simulink model "DR18E_Testpult"  (R2017a)
settings: Solver=ode1  StartTime=0.0  StopTime=Inf  FixedStep=0.001  RelTol=1e-3
PostLoadFcn:
  | , if any(exist('dsrtsu_mdlpostloadfcn', 'file') == [2, 3, 6]), try dsrtsu_mdlpostloadfcn('Execute', bdroot); catch fprintf('Error in PostLoadFcn (dsrtsu_mdlpostloadfcn) for model "%s":\n %s\n', bdroot, lasterr); end, end,
model workspace: external: MATLAB File C:\Users\DeltaRacing\Documents\dSPACE\MABX_DR18E\Model\DR18E_MABX_Parameter.m (data not in the file)
values from neighbouring files (symbols this model uses):
  am = 1/Ts    (= 1)    [DR18E_MABX_Parameter.m]
  bm = K/Ts    (= 0.05)    [DR18E_MABX_Parameter.m]
  cf = 41350    [DR18E_MABX_Parameter.m]
  cr = 41350    [DR18E_MABX_Parameter.m]
  Derating_HV_Battery_Kapa = 1    [DR18E_MABX_Parameter.m]
  Derating_Start_km = 16    [DR18E_MABX_Parameter.m]
  Drive_Mode = 0    [DR18E_MABX_Parameter.m]
  g = 1    [DR18E_MABX_Parameter.m]
  Gas_Modus = 2    [DR18E_MABX_Parameter.m]
  HV_Power_max = 80    [DR18E_MABX_Parameter.m]
  i_Getriebe = 3.3    [DR18E_MABX_Parameter.m]
  i_Lenkgetriebe = 4.32    [DR18E_MABX_Parameter.m]
  K_SET = 1    [DR18E_MABX_Parameter.m]
  Kapazitaet_HV_Battery_kWh = 6.6    [DR18E_MABX_Parameter.m]
  KW_T_Soll = 37    [DR18E_MABX_Parameter.m]
  lf = 1.2    [DR18E_MABX_Parameter.m]
  lr = 1.15    [DR18E_MABX_Parameter.m]
  m = 310    [DR18E_MABX_Parameter.m]
  M_max = 150    [DR18E_MABX_Parameter.m]
  Power_Limit_onoff = 0    [DR18E_MABX_Parameter.m]
  Reifenradius = 0.2351    [DR18E_MABX_Parameter.m]
  Strecke_Endu_km = 22    [DR18E_MABX_Parameter.m]
  TC_Decr_Gas = 0.00005    (= 5e-05)    [DR18E_MABX_Parameter.m]
  TC_Derivative = 0.4    [DR18E_MABX_Parameter.m]
  TC_Incr_Gas = 0.005    [DR18E_MABX_Parameter.m]
  TC_On = 0    [DR18E_MABX_Parameter.m]
  TC_Relay_Off = 0.065    [DR18E_MABX_Parameter.m]
  TC_Relay_On = 0.07    [DR18E_MABX_Parameter.m]
  TV_Mode = 2    [DR18E_MABX_Parameter.m]
  TV_On = 0    [DR18E_MABX_Parameter.m]
  TV_Override = 1    [DR18E_MABX_Parameter.m]
  y = 0.8    [DR18E_MABX_Parameter.m]
undefined symbols (not defined in the file or in its folder): D, DiscIntNeverNeededParam, I, K_OL, P
libraries: simulink x288, rtican x105, rtiusbflightreclib x40, rti1401lib_dio_type3 x10, simulink_extras x10, rti1401lib_adc_type4 x8, rti1401lib_II_base x7
(part 17 of 28)

== system DR18E_Testpult/Eingabe Fahrzeug/MicroAutoBox/Beschleunigungssensor ==
  Bus Creator : BusCreator  Inputs=3
  DS1401_ACCEL_READ_BL1 : rti1401lib_II_base/DS1401_ACCEL_READ_BL1  DSProperties=struct('RTI',struct('Version',uint32(1),'BlockType',struct('isSLSource',uint8(1),'isSLSink',uint8(0),'isHWSource',uint8(1),'isHWSink',uint8(0),'isSetup',uint8(0),'isInline',uint8(1),'isNonInline',uint8(0),'isInterrupt',uint8(0),'isChannelwise',uint8(0)),'IOBoardType',{{'DS1401','BASE','II'}},'UnitType','ACCEL','Identifier','ACCELREAD','DialogType','ML','BlockSet','NONE','SlaveProcessor','NONE'))  RTIBlockInterface=struct('OutputPortsWidth',int32([1 1 1 1]),'OutputPortsActive',[1 1 1 1],'OutputPortsDataType',{{'SS_UINT32','SS_DOUBLE','SS_DOUBLE','SS_DOUBLE'}},'OutputPortsName',{{'Count','X','Y','Z'}},'BlockDisplay',{{'Acceleration\nSensor','center'}},'IconTransparency','on','InitLevel',3,'DialogFcn','rti1401baseiiaccelreadgui','BlockName',struct('Token',{{'DS1401_ACCEL_READ_BL1'}}))  RTIBlockParameters=struct('SampleRate',{{5,'OFF',[1 8]}},'ReadMode',{{1,'OFF',[1 2]}},'SensorRange',{{3,'OFF',[1 3]}},'TLCFileName',{{'rti1401base_II_accel_read','OFF',[]}})  RTISFcnParameters=struct('SampleRate','int16','ReadMode','int16','SensorRange','int16','TLCFileName','char')  RTIBlockParaDefault=struct('SampleRate',3,'ReadMode',1,'SensorRange',1,'TLCFileName','rti1401base_II_accel_read')
  Beschleunigungssensor : Outport
  wires:
  Bus Creator/1 -> Beschleunigungssensor/1  "Beschleunigungssensor"
  DS1401_ACCEL_READ_BL1/2 -> Bus Creator/1  "x"
  DS1401_ACCEL_READ_BL1/3 -> Bus Creator/2  "y"
  DS1401_ACCEL_READ_BL1/4 -> Bus Creator/3  "z"

== system DR18E_Testpult/Eingabe Fahrzeug/MicroAutoBox/DI ==
  note: Direct DI
  note: Soundboard
  Bus Creator : BusCreator  Inputs=11
  DIO_TYPE3_BIT_IN_CH_BL1 : rti1401lib_dio_type3/DIO_TYPE3_BIT_IN_CH_BL1  DSProperties=struct('RTI',struct('Version',uint32(2),'BlockType',struct('isSLSource',uint8(1),'isSLSink',uint8(0),'isHWSource',uint8(1),'isHWSink',uint8(0),'isSetup',uint8(0),'isInline',uint8(1),'isNonInline',uint8(0),'isInterrupt',uint8(0),'isChannelwise',uint8(1)),'IOBoardType',{{'DS1401','STD','DIOT3'}},'UnitType','BIT','Identifier','BITINCH','DialogType','ML','BlockSet','NONE','SlaveProcessor','NONE'))  RTIBlockInterface=struct('OutputPortsWidth',int32(1),'OutputPortsDataType',{{'SS_BOOLEAN'}},'OutputPortsActive',1,'OutputPortsName',{{'Out'}},'BlockDisplay',{{['DIO TP3 BIT IN\n Channelwise\nModule: 1\nPort: 2\nChannel: 1'],'center'}},'IconTransparency','on','InitLevel',3,'DialogFcn','rti1401stddiot3bitinchgui','BlockName',struct('Token',{{'DIO_TYPE3_BIT_IN_CH_BL1'}}))  RTIBlockParameters=struct('ModuleNo',{{1,'OFF',[1 16]}},'PortNo',{{2,'OFF',[1 3]}},'ChannelNo',{{1,'OFF',[1 16]}},'TLCFileName',{{'rti1401dio_t3_bit_in_ch','OFF',[]}},'EnableInterrupt',{{0,'OFF',[0 1]}},'TriggerEdgeType',{{1,'OFF',[1 3]}})  RTISFcnParameters=struct('ModuleNo','int32','PortNo','int16','ChannelNo','int16','TLCFileName','char','EnableInterrupt','int16','TriggerEdgeType','int32')  RTIBlockParaDefault=struct('ModuleNo',1,'PortNo',1,'ChannelNo',1,'TLCFileName','rti1401dio_t3_bit_in_ch','EnableInterrupt',0,'TriggerEdgeType',1)
  DIO_TYPE3_BIT_IN_CH_BL10 : rti1401lib_dio_type3/DIO_TYPE3_BIT_IN_CH_BL1  DSProperties=struct('RTI',struct('Version',uint32(2),'BlockType',struct('isSLSource',uint8(1),'isSLSink',uint8(0),'isHWSource',uint8(1),'isHWSink',uint8(0),'isSetup',uint8(0),'isInline',uint8(1),'isNonInline',uint8(0),'isInterrupt',uint8(0),'isChannelwise',uint8(1)),'IOBoardType',{{'DS1401','STD','DIOT3'}},'UnitType','BIT','Identifier','BITINCH','DialogType','ML','BlockSet','NONE','SlaveProcessor','NONE'))  RTIBlockInterface=struct('OutputPortsWidth',int32(1),'OutputPortsDataType',{{'SS_BOOLEAN'}},'OutputPortsActive',1,'OutputPortsName',{{'Out'}},'BlockDisplay',{{['DIO TP3 BIT IN\n Channelwise\nModule: 1\nPort: 2\nChannel: 11'],'center'}},'IconTransparency','on','InitLevel',3,'DialogFcn','rti1401stddiot3bitinchgui','BlockName',struct('Token',{{'DIO_TYPE3_BIT_IN_CH_BL1'}}))  RTIBlockParameters=struct('ModuleNo',{{1,'OFF',[1 16]}},'PortNo',{{2,'OFF',[1 3]}},'ChannelNo',{{11,'OFF',[1 16]}},'TLCFileName',{{'rti1401dio_t3_bit_in_ch','OFF',[]}},'EnableInterrupt',{{0,'OFF',[0 1]}},'TriggerEdgeType',{{1,'OFF',[1 3]}})  RTISFcnParameters=struct('ModuleNo','int32','PortNo','int16','ChannelNo','int16','TLCFileName','char','EnableInterrupt','int16','TriggerEdgeType','int32')  RTIBlockParaDefault=struct('ModuleNo',1,'PortNo',1,'ChannelNo',1,'TLCFileName','rti1401dio_t3_bit_in_ch','EnableInterrupt',0,'TriggerEdgeType',1)
  DIO_TYPE3_BIT_IN_CH_BL2 : rti1401lib_dio_type3/DIO_TYPE3_BIT_IN_CH_BL1  DSProperties=struct('RTI',struct('Version',uint32(2),'BlockType',struct('isSLSource',uint8(1),'isSLSink',uint8(0),'isHWSource',uint8(1),'isHWSink',uint8(0),'isSetup',uint8(0),'isInline',uint8(1),'isNonInline',uint8(0),'isInterrupt',uint8(0),'isChannelwise',uint8(1)),'IOBoardType',{{'DS1401','STD','DIOT3'}},'UnitType','BIT','Identifier','BITINCH','DialogType','ML','BlockSet','NONE','SlaveProcessor','NONE'))  RTIBlockInterface=struct('OutputPortsWidth',int32(1),'OutputPortsDataType',{{'SS_BOOLEAN'}},'OutputPortsActive',1,'OutputPortsName',{{'Out'}},'BlockDisplay',{{['DIO TP3 BIT IN\n Channelwise\nModule: 1\nPort: 2\nChannel: 2'],'center'}},'IconTransparency','on','InitLevel',3,'DialogFcn','rti1401stddiot3bitinchgui','BlockName',struct('Token',{{'DIO_TYPE3_BIT_IN_CH_BL1'}}))  RTIBlockParameters=struct('ModuleNo',{{1,'OFF',[1 16]}},'PortNo',{{2,'OFF',[1 3]}},'ChannelNo',{{2,'OFF',[1 16]}},'TLCFileName',{{'rti1401dio_t3_bit_in_ch','OFF',[]}},'EnableInterrupt',{{0,'OFF',[0 1]}},'TriggerEdgeType',{{1,'OFF',[1 3]}})  RTISFcnParameters=struct('ModuleNo','int32','PortNo','int16','ChannelNo','int16','TLCFileName','char','EnableInterrupt','int16','TriggerEdgeType','int32')  RTIBlockParaDefault=struct('ModuleNo',1,'PortNo',1,'ChannelNo',1,'TLCFileName','rti1401dio_t3_bit_in_ch','EnableInterrupt',0,'TriggerEdgeType',1)
  DIO_TYPE3_BIT_IN_CH_BL3 : rti1401lib_dio_type3/DIO_TYPE3_BIT_IN_CH_BL1  DSProperties=struct('RTI',struct('Version',uint32(2),'BlockType',struct('isSLSource',uint8(1),'isSLSink',uint8(0),'isHWSource',uint8(1),'isHWSink',uint8(0),'isSetup',uint8(0),'isInline',uint8(1),'isNonInline',uint8(0),'isInterrupt',uint8(0),'isChannelwise',uint8(1)),'IOBoardType',{{'DS1401','STD','DIOT3'}},'UnitType','BIT','Identifier','BITINCH','DialogType','ML','BlockSet','NONE','SlaveProcessor','NONE'))  RTIBlockInterface=struct('OutputPortsWidth',int32(1),'OutputPortsDataType',{{'SS_BOOLEAN'}},'OutputPortsActive',1,'OutputPortsName',{{'Out'}},'BlockDisplay',{{['DIO TP3 BIT IN\n Channelwise\nModule: 1\nPort: 2\nChannel: 6'],'center'}},'IconTransparency','on','InitLevel',3,'DialogFcn','rti1401stddiot3bitinchgui','BlockName',struct('Token',{{'DIO_TYPE3_BIT_IN_CH_BL1'}}))  RTIBlockParameters=struct('ModuleNo',{{1,'OFF',[1 16]}},'PortNo',{{2,'OFF',[1 3]}},'ChannelNo',{{6,'OFF',[1 16]}},'TLCFileName',{{'rti1401dio_t3_bit_in_ch','OFF',[]}},'EnableInterrupt',{{0,'OFF',[0 1]}},'TriggerEdgeType',{{1,'OFF',[1 3]}})  RTISFcnParameters=struct('ModuleNo','int32','PortNo','int16','ChannelNo','int16','TLCFileName','char','EnableInterrupt','int16','TriggerEdgeType','int32')  RTIBlockParaDefault=struct('ModuleNo',1,'PortNo',1,'ChannelNo',1,'TLCFileName','rti1401dio_t3_bit_in_ch','EnableInterrupt',0,'TriggerEdgeType',1)
  DIO_TYPE3_BIT_IN_CH_BL4 : rti1401lib_dio_type3/DIO_TYPE3_BIT_IN_CH_BL1  DSProperties=struct('RTI',struct('Version',uint32(2),'BlockType',struct('isSLSource',uint8(1),'isSLSink',uint8(0),'isHWSource',uint8(1),'isHWSink',uint8(0),'isSetup',uint8(0),'isInline',uint8(1),'isNonInline',uint8(0),'isInterrupt',uint8(0),'isChannelwise',uint8(1)),'IOBoardType',{{'DS1401','STD','DIOT3'}},'UnitType','BIT','Identifier','BITINCH','DialogType','ML','BlockSet','NONE','SlaveProcessor','NONE'))  RTIBlockInterface=struct('OutputPortsWidth',int32(1),'OutputPortsDataType',{{'SS_BOOLEAN'}},'OutputPortsActive',1,'OutputPortsName',{{'Out'}},'BlockDisplay',{{['DIO TP3 BIT IN\n Channelwise\nModule: 1\nPort: 2\nChannel: 4'],'center'}},'IconTransparency','on','InitLevel',3,'DialogFcn','rti1401stddiot3bitinchgui','BlockName',struct('Token',{{'DIO_TYPE3_BIT_IN_CH_BL1'}}))  RTIBlockParameters=struct('ModuleNo',{{1,'OFF',[1 16]}},'PortNo',{{2,'OFF',[1 3]}},'ChannelNo',{{4,'OFF',[1 16]}},'TLCFileName',{{'rti1401dio_t3_bit_in_ch','OFF',[]}},'EnableInterrupt',{{0,'OFF',[0 1]}},'TriggerEdgeType',{{1,'OFF',[1 3]}})  RTISFcnParameters=struct('ModuleNo','int32','PortNo','int16','ChannelNo','int16','TLCFileName','char','EnableInterrupt','int16','TriggerEdgeType','int32')  RTIBlockParaDefault=struct('ModuleNo',1,'PortNo',1,'ChannelNo',1,'TLCFileName','rti1401dio_t3_bit_in_ch','EnableInterrupt',0,'TriggerEdgeType',1)
  DIO_TYPE3_BIT_IN_CH_BL5 : rti1401lib_dio_type3/DIO_TYPE3_BIT_IN_CH_BL1  DSProperties=struct('RTI',struct('Version',uint32(2),'BlockType',struct('isSLSource',uint8(1),'isSLSink',uint8(0),'isHWSource',uint8(1),'isHWSink',uint8(0),'isSetup',uint8(0),'isInline',uint8(1),'isNonInline',uint8(0),'isInterrupt',uint8(0),'isChannelwise',uint8(1)),'IOBoardType',{{'DS1401','STD','DIOT3'}},'UnitType','BIT','Identifier','BITINCH','DialogType','ML','BlockSet','NONE','SlaveProcessor','NONE'))  RTIBlockInterface=struct('OutputPortsWidth',int32(1),'OutputPortsDataType',{{'SS_BOOLEAN'}},'OutputPortsActive',1,'OutputPortsName',{{'Out'}},'BlockDisplay',{{['DIO TP3 BIT IN\n Channelwise\nModule: 1\nPort: 2\nChannel: 5'],'center'}},'IconTransparency','on','InitLevel',3,'DialogFcn','rti1401stddiot3bitinchgui','BlockName',struct('Token',{{'DIO_TYPE3_BIT_IN_CH_BL1'}}))  RTIBlockParameters=struct('ModuleNo',{{1,'OFF',[1 16]}},'PortNo',{{2,'OFF',[1 3]}},'ChannelNo',{{5,'OFF',[1 16]}},'TLCFileName',{{'rti1401dio_t3_bit_in_ch','OFF',[]}},'EnableInterrupt',{{0,'OFF',[0 1]}},'TriggerEdgeType',{{1,'OFF',[1 3]}})  RTISFcnParameters=struct('ModuleNo','int32','PortNo','int16','ChannelNo','int16','TLCFileName','char','EnableInterrupt','int16','TriggerEdgeType','int32')  RTIBlockParaDefault=struct('ModuleNo',1,'PortNo',1,'ChannelNo',1,'TLCFileName','rti1401dio_t3_bit_in_ch','EnableInterrupt',0,'TriggerEdgeType',1)
  DIO_TYPE3_BIT_IN_CH_BL6 : rti1401lib_dio_type3/DIO_TYPE3_BIT_IN_CH_BL1  DSProperties=struct('RTI',struct('Version',uint32(2),'BlockType',struct('isSLSource',uint8(1),'isSLSink',uint8(0),'isHWSource',uint8(1),'isHWSink',uint8(0),'isSetup',uint8(0),'isInline',uint8(1),'isNonInline',uint8(0),'isInterrupt',uint8(0),'isChannelwise',uint8(1)),'IOBoardType',{{'DS1401','STD','DIOT3'}},'UnitType','BIT','Identifier','BITINCH','DialogType','ML','BlockSet','NONE','SlaveProcessor','NONE'))  RTIBlockInterface=struct('OutputPortsWidth',int32(1),'OutputPortsDataType',{{'SS_BOOLEAN'}},'OutputPortsActive',1,'OutputPortsName',{{'Out'}},'BlockDisplay',{{['DIO TP3 BIT IN\n Channelwise\nModule: 1\nPort: 2\nChannel: 8'],'center'}},'IconTransparency','on','InitLevel',3,'DialogFcn','rti1401stddiot3bitinchgui','BlockName',struct('Token',{{'DIO_TYPE3_BIT_IN_CH_BL1'}}))  RTIBlockParameters=struct('ModuleNo',{{1,'OFF',[1 16]}},'PortNo',{{2,'OFF',[1 3]}},'ChannelNo',{{8,'OFF',[1 16]}},'TLCFileName',{{'rti1401dio_t3_bit_in_ch','OFF',[]}},'EnableInterrupt',{{0,'OFF',[0 1]}},'TriggerEdgeType',{{1,'OFF',[1 3]}})  RTISFcnParameters=struct('ModuleNo','int32','PortNo','int16','ChannelNo','int16','TLCFileName','char','EnableInterrupt','int16','TriggerEdgeType','int32')  RTIBlockParaDefault=struct('ModuleNo',1,'PortNo',1,'ChannelNo',1,'TLCFileName','rti1401dio_t3_bit_in_ch','EnableInterrupt',0,'TriggerEdgeType',1)
  DIO_TYPE3_BIT_IN_CH_BL7 : rti1401lib_dio_type3/DIO_TYPE3_BIT_IN_CH_BL1  DSProperties=struct('RTI',struct('Version',uint32(2),'BlockType',struct('isSLSource',uint8(1),'isSLSink',uint8(0),'isHWSource',uint8(1),'isHWSink',uint8(0),'isSetup',uint8(0),'isInline',uint8(1),'isNonInline',uint8(0),'isInterrupt',uint8(0),'isChannelwise',uint8(1)),'IOBoardType',{{'DS1401','STD','DIOT3'}},'UnitType','BIT','Identifier','BITINCH','DialogType','ML','BlockSet','NONE','SlaveProcessor','NONE'))  RTIBlockInterface=struct('OutputPortsWidth',int32(1),'OutputPortsDataType',{{'SS_BOOLEAN'}},'OutputPortsActive',1,'OutputPortsName',{{'Out'}},'BlockDisplay',{{['DIO TP3 BIT IN\n Channelwise\nModule: 1\nPort: 2\nChannel: 9'],'center'}},'IconTransparency','on','InitLevel',3,'DialogFcn','rti1401stddiot3bitinchgui','BlockName',struct('Token',{{'DIO_TYPE3_BIT_IN_CH_BL1'}}))  RTIBlockParameters=struct('ModuleNo',{{1,'OFF',[1 16]}},'PortNo',{{2,'OFF',[1 3]}},'ChannelNo',{{9,'OFF',[1 16]}},'TLCFileName',{{'rti1401dio_t3_bit_in_ch','OFF',[]}},'EnableInterrupt',{{0,'OFF',[0 1]}},'TriggerEdgeType',{{1,'OFF',[1 3]}})  RTISFcnParameters=struct('ModuleNo','int32','PortNo','int16','ChannelNo','int16','TLCFileName','char','EnableInterrupt','int16','TriggerEdgeType','int32')  RTIBlockParaDefault=struct('ModuleNo',1,'PortNo',1,'ChannelNo',1,'TLCFileName','rti1401dio_t3_bit_in_ch','EnableInterrupt',0,'TriggerEdgeType',1)
  DIO_TYPE3_BIT_IN_CH_BL8 : rti1401lib_dio_type3/DIO_TYPE3_BIT_IN_CH_BL1  DSProperties=struct('RTI',struct('Version',uint32(2),'BlockType',struct('isSLSource',uint8(1),'isSLSink',uint8(0),'isHWSource',uint8(1),'isHWSink',uint8(0),'isSetup',uint8(0),'isInline',uint8(1),'isNonInline',uint8(0),'isInterrupt',uint8(0),'isChannelwise',uint8(1)),'IOBoardType',{{'DS1401','STD','DIOT3'}},'UnitType','BIT','Identifier','BITINCH','DialogType','ML','BlockSet','NONE','SlaveProcessor','NONE'))  RTIBlockInterface=struct('OutputPortsWidth',int32(1),'OutputPortsDataType',{{'SS_BOOLEAN'}},'OutputPortsActive',1,'OutputPortsName',{{'Out'}},'BlockDisplay',{{['DIO TP3 BIT IN\n Channelwise\nModule: 1\nPort: 2\nChannel: 10'],'center'}},'IconTransparency','on','InitLevel',3,'DialogFcn','rti1401stddiot3bitinchgui','BlockName',struct('Token',{{'DIO_TYPE3_BIT_IN_CH_BL1'}}))  RTIBlockParameters=struct('ModuleNo',{{1,'OFF',[1 16]}},'PortNo',{{2,'OFF',[1 3]}},'ChannelNo',{{10,'OFF',[1 16]}},'TLCFileName',{{'rti1401dio_t3_bit_in_ch','OFF',[]}},'EnableInterrupt',{{0,'OFF',[0 1]}},'TriggerEdgeType',{{1,'OFF',[1 3]}})  RTISFcnParameters=struct('ModuleNo','int32','PortNo','int16','ChannelNo','int16','TLCFileName','char','EnableInterrupt','int16','TriggerEdgeType','int32')  RTIBlockParaDefault=struct('ModuleNo',1,'PortNo',1,'ChannelNo',1,'TLCFileName','rti1401dio_t3_bit_in_ch','EnableInterrupt',0,'TriggerEdgeType',1)
  DIO_TYPE3_BIT_IN_CH_BL9 : rti1401lib_dio_type3/DIO_TYPE3_BIT_IN_CH_BL1  DSProperties=struct('RTI',struct('Version',uint32(2),'BlockType',struct('isSLSource',uint8(1),'isSLSink',uint8(0),'isHWSource',uint8(1),'isHWSink',uint8(0),'isSetup',uint8(0),'isInline',uint8(1),'isNonInline',uint8(0),'isInterrupt',uint8(0),'isChannelwise',uint8(1)),'IOBoardType',{{'DS1401','STD','DIOT3'}},'UnitType','BIT','Identifier','BITINCH','DialogType','ML','BlockSet','NONE','SlaveProcessor','NONE'))  RTIBlockInterface=struct('OutputPortsWidth',int32(1),'OutputPortsDataType',{{'SS_BOOLEAN'}},'OutputPortsActive',1,'OutputPortsName',{{'Out'}},'BlockDisplay',{{['DIO TP3 BIT IN\n Channelwise\nModule: 1\nPort: 2\nChannel: 7'],'center'}},'IconTransparency','on','InitLevel',3,'DialogFcn','rti1401stddiot3bitinchgui','BlockName',struct('Token',{{'DIO_TYPE3_BIT_IN_CH_BL1'}}))  RTIBlockParameters=struct('ModuleNo',{{1,'OFF',[1 16]}},'PortNo',{{2,'OFF',[1 3]}},'ChannelNo',{{7,'OFF',[1 16]}},'TLCFileName',{{'rti1401dio_t3_bit_in_ch','OFF',[]}},'EnableInterrupt',{{0,'OFF',[0 1]}},'TriggerEdgeType',{{1,'OFF',[1 3]}})  RTISFcnParameters=struct('ModuleNo','int32','PortNo','int16','ChannelNo','int16','TLCFileName','char','EnableInterrupt','int16','TriggerEdgeType','int32')  RTIBlockParaDefault=struct('ModuleNo',1,'PortNo',1,'ChannelNo',1,'TLCFileName','rti1401dio_t3_bit_in_ch','EnableInterrupt',0,'TriggerEdgeType',1)
  DI : Outport
  wires:
  Bus Creator/1 -> DI/1  "DI"
  DIO_TYPE3_BIT_IN_CH_BL1/1 -> Bus Creator/1  "DI8_P2Ch1"
  DIO_TYPE3_BIT_IN_CH_BL2/1 -> Bus Creator/2  "DI7_P2Ch2"
  DIO_TYPE3_BIT_IN_CH_BL4/1 -> Bus Creator/4  "DI5_P2Ch4_AIR1"
  DIO_TYPE3_BIT_IN_CH_BL5/1 -> Bus Creator/5  "DI4_P2Ch5_AIR2"
  DIO_TYPE3_BIT_IN_CH_BL7/1 -> Bus Creator/7  "DI2_P2Ch9_AIR4"
  DIO_TYPE3_BIT_IN_CH_BL8/1 -> Bus Creator/8  "DI1_P2Ch10_Crash"
  DIO_TYPE3_BIT_IN_CH_BL9/1 -> Bus Creator/9  "P2Ch7_IMDAMS_Reset"
  DIO_TYPE3_BIT_IN_CH_BL6/1 -> Bus Creator/10  "P2Ch8_NotausLinks"
  DIO_TYPE3_BIT_IN_CH_BL10/1 -> Bus Creator/11  "P2Ch11_NotausRechts"
  DIO_TYPE3_BIT_IN_CH_BL3/1 -> Bus Creator/6  "DI3_P2Ch6_AIR3"

== system DR18E_Testpult/Eingabe Fahrzeug/Sensorboard Front/RX OK Detection1 ==
  note: This subsystem surveys if the sending of the TX message is successful and if it meets the
      | requirements concerning the regularity of the sending.
      |
      | If for 5 consecutive execution steps the message could not be successfully sent the 'TX Warn'
      | output is set to 1. Also, the message is expected to be sent every 50 ms approximatively. If this
      | condition is not met 5 times consecutively the 'TX Warn' output is set to 1.
  TX status : Inport
  TX delta time : Inport  Port=2
  Delta time limit : Constant  Value=0.055
  Delta time limit exceeded : RelationalOperator  RndMeth=Nearest  InputSameDT=on
  Mem{1..4} (4 alike) : Memory
  OR : Logic  Operator=OR
  Prev. msg. not sent : RelationalOperator  Operator=~=  RndMeth=Nearest  InputSameDT=on
  Prev. msg. sent value : Constant
  Warn : Logic  Inputs=5
  TX Warn : Outport
  wires:
  TX delta time/1 -> Delta time limit exceeded/1
  Delta time limit/1 -> Delta time limit exceeded/2
  Prev. msg. sent value/1 -> Prev. msg. not sent/2
  TX status/1 -> Prev. msg. not sent/1
  Prev. msg. not sent/1 -> OR/1
  Delta time limit exceeded/1 -> OR/2
  OR/1 -> Mem1/1, Warn/1
  Mem1/1 -> Mem2/1, Warn/2
  Mem2/1 -> Mem3/1, Warn/3
  Mem3/1 -> Mem4/1, Warn/4
  Mem4/1 -> Warn/5
  Warn/1 -> TX Warn/1

== system DR18E_Testpult/Eingabe Fahrzeug/Sensorboard Front/RX OK Detection3 ==
  note: This subsystem surveys if the sending of the TX message is successful and if it meets the
      | requirements concerning the regularity of the sending.
      |
      | If for 5 consecutive execution steps the message could not be successfully sent the 'TX Warn'
      | output is set to 1. Also, the message is expected to be sent every 50 ms approximatively. If this
      | condition is not met 5 times consecutively the 'TX Warn' output is set to 1.
  TX status : Inport
  TX delta time : Inport  Port=2
  Delta time limit : Constant  Value=0.055
  Delta time limit exceeded : RelationalOperator  RndMeth=Nearest  InputSameDT=on
  Mem{1..4} (4 alike) : Memory
  OR : Logic  Operator=OR
  Prev. msg. not sent : RelationalOperator  Operator=~=  RndMeth=Nearest  InputSameDT=on
  Prev. msg. sent value : Constant
  Warn : Logic  Inputs=5
  TX Warn : Outport
  wires:
  TX delta time/1 -> Delta time limit exceeded/1
  Delta time limit/1 -> Delta time limit exceeded/2
  Prev. msg. sent value/1 -> Prev. msg. not sent/2
  TX status/1 -> Prev. msg. not sent/1
  Prev. msg. not sent/1 -> OR/1
  Delta time limit exceeded/1 -> OR/2
  OR/1 -> Mem1/1, Warn/1
  Mem1/1 -> Mem2/1, Warn/2
  Mem2/1 -> Mem3/1, Warn/3
  Mem3/1 -> Mem4/1, Warn/4
  Mem4/1 -> Warn/5
  Warn/1 -> TX Warn/1

== system DR18E_Testpult/Eingabe Fahrzeug/Sensorboard Front/RX OK Detection4 ==
  note: This subsystem surveys if the sending of the TX message is successful and if it meets the
      | requirements concerning the regularity of the sending.
      |
      | If for 5 consecutive execution steps the message could not be successfully sent the 'TX Warn'
      | output is set to 1. Also, the message is expected to be sent every 50 ms approximatively. If this
      | condition is not met 5 times consecutively the 'TX Warn' output is set to 1.
  TX status : Inport
  TX delta time : Inport  Port=2
  Delta time limit : Constant  Value=0.055
  Delta time limit exceeded : RelationalOperator  RndMeth=Nearest  InputSameDT=on
  Mem{1..4} (4 alike) : Memory
  OR : Logic  Operator=OR
  Prev. msg. not sent : RelationalOperator  Operator=~=  RndMeth=Nearest  InputSameDT=on
  Prev. msg. sent value : Constant
  Warn : Logic  Inputs=5
  TX Warn : Outport
  wires:
  TX delta time/1 -> Delta time limit exceeded/1
  Delta time limit/1 -> Delta time limit exceeded/2
  Prev. msg. sent value/1 -> Prev. msg. not sent/2
  TX status/1 -> Prev. msg. not sent/1
  Prev. msg. not sent/1 -> OR/1
  Delta time limit exceeded/1 -> OR/2
  OR/1 -> Mem1/1, Warn/1
  Mem1/1 -> Mem2/1, Warn/2
  Mem2/1 -> Mem3/1, Warn/3
  Mem3/1 -> Mem4/1, Warn/4
  Mem4/1 -> Warn/5
  Warn/1 -> TX Warn/1

== system DR18E_Testpult/Eingabe Fahrzeug/Sensorboard Front/RX Timeout Detection ==
  RX status : Inport
  Timeout (n Samples) : Inport  Port=2
  Terminator_4 : Terminator
  Triggered Subsystem : Subsystem  TreatAsAtomicUnit=on
  RX Timeout Error : Outport
  wires:
  RX status/1 -> Triggered Subsystem/1(TXStatus)
  Triggered Subsystem/1(Rampe) -> Terminator_4/1
  Triggered Subsystem/2(RX Timeout Error) -> RX Timeout Error/1  "RX Timeout"
  Timeout (n Samples)/1 -> Triggered Subsystem/2(Timeout)

== system DR18E_Testpult/Eingabe Fahrzeug/Sensorboard Front/RX Timeout Detection1 ==
  RX status : Inport
  Timeout (n Samples) : Inport  Port=2
  Terminator_4 : Terminator
  Triggered Subsystem : Subsystem  TreatAsAtomicUnit=on
  RX Timeout Error : Outport
  wires:
  RX status/1 -> Triggered Subsystem/1(TXStatus)
  Triggered Subsystem/1(Rampe) -> Terminator_4/1
  Triggered Subsystem/2(RX Timeout Error) -> RX Timeout Error/1  "RX Timeout"
  Timeout (n Samples)/1 -> Triggered Subsystem/2(Timeout)

== system DR18E_Testpult/Eingabe Fahrzeug/Sensorboard Mitte/RX Timeout Detection ==
  RX status : Inport
  Timeout (n Samples) : Inport  Port=2
  Terminator_4 : Terminator
  Triggered Subsystem : Subsystem  TreatAsAtomicUnit=on
  RX Timeout Error : Outport
  wires:
  RX status/1 -> Triggered Subsystem/1(TXStatus)
  Triggered Subsystem/1(Rampe) -> Terminator_4/1
  Triggered Subsystem/2(RX Timeout Error) -> RX Timeout Error/1  "RX Timeout"
  Timeout (n Samples)/1 -> Triggered Subsystem/2(Timeout)

== system DR18E_Testpult/Eingabe Fahrzeug/Sensorboard Mitte/Transmit OK Detection3 ==
  note: This subsystem surveys if the sending of the TX message is successful and if it meets the
      | requirements concerning the regularity of the sending.
      |
      | If for 5 consecutive execution steps the message could not be successfully sent the 'TX Warn'
      | output is set to 1. Also, the message is expected to be sent every 50 ms approximatively. If this
      | condition is not met 5 times consecutively the 'TX Warn' output is set to 1.
  TX status : Inport
  TX delta time : Inport  Port=2
  Delta time limit : Constant  Value=0.055
  Delta time limit exceeded : RelationalOperator  RndMeth=Nearest  InputSameDT=on
  Mem{1..4} (4 alike) : Memory
  OR : Logic  Operator=OR
  Prev. msg. not sent : RelationalOperator  Operator=~=  RndMeth=Nearest  InputSameDT=on
  Prev. msg. sent value : Constant
  Warn : Logic  Inputs=5
  TX Warn : Outport
  wires:
  TX delta time/1 -> Delta time limit exceeded/1
  Delta time limit/1 -> Delta time limit exceeded/2
  Prev. msg. sent value/1 -> Prev. msg. not sent/2
  TX status/1 -> Prev. msg. not sent/1
  Prev. msg. not sent/1 -> OR/1
  Delta time limit exceeded/1 -> OR/2
  OR/1 -> Mem1/1, Warn/1
  Mem1/1 -> Mem2/1, Warn/2
  Mem2/1 -> Mem3/1, Warn/3
  Mem3/1 -> Mem4/1, Warn/4
  Mem4/1 -> Warn/5
  Warn/1 -> TX Warn/1

== system DR18E_Testpult/Eingabe Fahrzeug/Sensorboard Mitte/Transmit OK Detection4 ==
  note: This subsystem surveys if the sending of the TX message is successful and if it meets the
      | requirements concerning the regularity of the sending.
      |
      | If for 5 consecutive execution steps the message could not be successfully sent the 'TX Warn'
      | output is set to 1. Also, the message is expected to be sent every 50 ms approximatively. If this
      | condition is not met 5 times consecutively the 'TX Warn' output is set to 1.
  TX status : Inport
  TX delta time : Inport  Port=2
  Delta time limit : Constant  Value=0.055
  Delta time limit exceeded : RelationalOperator  RndMeth=Nearest  InputSameDT=on
  Mem{1..4} (4 alike) : Memory
  OR : Logic  Operator=OR
  Prev. msg. not sent : RelationalOperator  Operator=~=  RndMeth=Nearest  InputSameDT=on
  Prev. msg. sent value : Constant
  Warn : Logic  Inputs=5
  TX Warn : Outport
  wires:
  TX delta time/1 -> Delta time limit exceeded/1
  Delta time limit/1 -> Delta time limit exceeded/2
  Prev. msg. sent value/1 -> Prev. msg. not sent/2
  TX status/1 -> Prev. msg. not sent/1
  Prev. msg. not sent/1 -> OR/1
  Delta time limit exceeded/1 -> OR/2
  OR/1 -> Mem1/1, Warn/1
  Mem1/1 -> Mem2/1, Warn/2
  Mem2/1 -> Mem3/1, Warn/3
  Mem3/1 -> Mem4/1, Warn/4
  Mem4/1 -> Warn/5
  Warn/1 -> TX Warn/1

== system DR18E_Testpult/Eingabe Fahrzeug/Sensorboard Rear/FlightRecorder1 ==
  In1 : Inport
  Data Type Conversion : DataTypeConversion
  Gain : Gain
  USB_FLIGHT_REC_BL1 : rtiusbflightreclib/USB_FLIGHT_REC_BL1  VarName=WaterPump  DataType=Single  SampleTime=0.5  TLCFileName=rtiusbflightrecwrite  Reserved1=[]  Reserved2=[]  Reserved3=[]  Reserved4=[]  DSProperties=struct('RTI',struct('Version',uint32(3),'BlockType',struct('isSLSource',uint8(0),'isSLSink',uint8(1),'isHWSource',uint8(0),'isHWSink',uint8(0),'isSetup',uint8(0),'isInline',uint8(1),'isNonInline',uint8(0),'isInterrupt',uint8(0),'isChannelwise',uint8(0)),'IOBoardType',{{'DSUSB','FLIGHTREC'}},'UnitType','FLIGHTREC','Identifier','WRITE','DialogType','SL','BlockSet','RTIUSBFLIGHTREC','SlaveProcessor','NONE'))  RTIBlockInterface=struct('InputPortsActive',1,'InputPortsWidth',int32(1),'InputPortsDataType',{{'SS_SINGLE'}},'BlockDisplay',{{['Write to\nUSB Flight Recorder'],'center'}},'IconTransparency','off','InitLevel',3,'BlockName',struct('Token',{{'USB_FLIGHT_REC_BL1'}}),'MaskDescription',['Write input to the Flight Recorder. Recorded data can be referenced by the specified variable.'],'SampleTime',{{2^-1}})  RTIBlockParameters=struct('VarName',{{'WaterPump','OFF',[]}},'DataType',{{'Single','OFF',[]}},'SampleTime',{{2^-1,'OFF',[]}},'TLCFileName',{{'rtiusbflightrecwrite','OFF',[]}})  RTISFcnParameters=struct('VarName','char','DataType','char','SampleTime','double','TLCFileName','char')  RTIBlockParaDefault=struct('VarName','Var1','DataType','Single','SampleTime',-1,'TLCFileName','rtiusbflightrecwrite')
      settings: SourceProductName=dSPACE RTI USB Flight Rec Blockset
  wires:
  Data Type Conversion/1 -> USB_FLIGHT_REC_BL1/1
  In1/1 -> Gain/1
  Gain/1 -> Data Type Conversion/1

== system DR18E_Testpult/Eingabe Fahrzeug/Sensorboard Rear/FlightRecorder2 ==
  In1 : Inport
  Data Type Conversion : DataTypeConversion
  Gain : Gain
  USB_FLIGHT_REC_BL1 : rtiusbflightreclib/USB_FLIGHT_REC_BL1  VarName=WaterCooler  DataType=Single  SampleTime=0.5  TLCFileName=rtiusbflightrecwrite  Reserved1=[]  Reserved2=[]  Reserved3=[]  Reserved4=[]  DSProperties=struct('RTI',struct('Version',uint32(3),'BlockType',struct('isSLSource',uint8(0),'isSLSink',uint8(1),'isHWSource',uint8(0),'isHWSink',uint8(0),'isSetup',uint8(0),'isInline',uint8(1),'isNonInline',uint8(0),'isInterrupt',uint8(0),'isChannelwise',uint8(0)),'IOBoardType',{{'DSUSB','FLIGHTREC'}},'UnitType','FLIGHTREC','Identifier','WRITE','DialogType','SL','BlockSet','RTIUSBFLIGHTREC','SlaveProcessor','NONE'))  RTIBlockInterface=struct('InputPortsActive',1,'InputPortsWidth',int32(1),'InputPortsDataType',{{'SS_SINGLE'}},'BlockDisplay',{{['Write to\nUSB Flight Recorder'],'center'}},'IconTransparency','off','InitLevel',3,'BlockName',struct('Token',{{'USB_FLIGHT_REC_BL1'}}),'MaskDescription',['Write input to the Flight Recorder. Recorded data can be referenced by the specified variable.'],'SampleTime',{{2^-1}})  RTIBlockParameters=struct('VarName',{{'WaterCooler','OFF',[]}},'DataType',{{'Single','OFF',[]}},'SampleTime',{{2^-1,'OFF',[]}},'TLCFileName',{{'rtiusbflightrecwrite','OFF',[]}})  RTISFcnParameters=struct('VarName','char','DataType','char','SampleTime','double','TLCFileName','char')  RTIBlockParaDefault=struct('VarName','Var1','DataType','Single','SampleTime',-1,'TLCFileName','rtiusbflightrecwrite')
      settings: SourceProductName=dSPACE RTI USB Flight Rec Blockset
  wires:
  Data Type Conversion/1 -> USB_FLIGHT_REC_BL1/1
  In1/1 -> Gain/1
  Gain/1 -> Data Type Conversion/1

== system DR18E_Testpult/Eingabe Fahrzeug/Sensorboard Rear/FlightRecorder3 ==
  In1 : Inport
  Data Type Conversion : DataTypeConversion
  Gain : Gain
  USB_FLIGHT_REC_BL1 : rtiusbflightreclib/USB_FLIGHT_REC_BL1  VarName=oiltemp  DataType=Single  SampleTime=0.5  TLCFileName=rtiusbflightrecwrite  Reserved1=[]  Reserved2=[]  Reserved3=[]  Reserved4=[]  DSProperties=struct('RTI',struct('Version',uint32(3),'BlockType',struct('isSLSource',uint8(0),'isSLSink',uint8(1),'isHWSource',uint8(0),'isHWSink',uint8(0),'isSetup',uint8(0),'isInline',uint8(1),'isNonInline',uint8(0),'isInterrupt',uint8(0),'isChannelwise',uint8(0)),'IOBoardType',{{'DSUSB','FLIGHTREC'}},'UnitType','FLIGHTREC','Identifier','WRITE','DialogType','SL','BlockSet','RTIUSBFLIGHTREC','SlaveProcessor','NONE'))  RTIBlockInterface=struct('InputPortsActive',1,'InputPortsWidth',int32(1),'InputPortsDataType',{{'SS_SINGLE'}},'BlockDisplay',{{['Write to\nUSB Flight Recorder'],'center'}},'IconTransparency','off','InitLevel',3,'BlockName',struct('Token',{{'USB_FLIGHT_REC_BL1'}}),'MaskDescription',['Write input to the Flight Recorder. Recorded data can be referenced by the specified variable.'],'SampleTime',{{2^-1}})  RTIBlockParameters=struct('VarName',{{'oiltemp','OFF',[]}},'DataType',{{'Single','OFF',[]}},'SampleTime',{{2^-1,'OFF',[]}},'TLCFileName',{{'rtiusbflightrecwrite','OFF',[]}})  RTISFcnParameters=struct('VarName','char','DataType','char','SampleTime','double','TLCFileName','char')  RTIBlockParaDefault=struct('VarName','Var1','DataType','Single','SampleTime',-1,'TLCFileName','rtiusbflightrecwrite')
      settings: SourceProductName=dSPACE RTI USB Flight Rec Blockset
  wires:
  Data Type Conversion/1 -> USB_FLIGHT_REC_BL1/1
  In1/1 -> Gain/1
  Gain/1 -> Data Type Conversion/1

== system DR18E_Testpult/Eingabe Fahrzeug/Sensorboard Rear/Transmit OK Detection1 ==
  note: This subsystem surveys if the sending of the TX message is successful and if it meets the
      | requirements concerning the regularity of the sending.
      |
      | If for 5 consecutive execution steps the message could not be successfully sent the 'TX Warn'
      | output is set to 1. Also, the message is expected to be sent every 50 ms approximatively. If this
      | condition is not met 5 times consecutively the 'TX Warn' output is set to 1.
  TX status : Inport
  TX delta time : Inport  Port=2
  Delta time limit : Constant  Value=0.055
  Delta time limit exceeded : RelationalOperator  RndMeth=Nearest  InputSameDT=on
  Mem{1..4} (4 alike) : Memory
  OR : Logic  Operator=OR
  Prev. msg. not sent : RelationalOperator  Operator=~=  RndMeth=Nearest  InputSameDT=on
  Prev. msg. sent value : Constant
  Warn : Logic  Inputs=5
  TX Warn : Outport
  wires:
  TX delta time/1 -> Delta time limit exceeded/1
  Delta time limit/1 -> Delta time limit exceeded/2
  Prev. msg. sent value/1 -> Prev. msg. not sent/2
  TX status/1 -> Prev. msg. not sent/1
  Prev. msg. not sent/1 -> OR/1
  Delta time limit exceeded/1 -> OR/2
  OR/1 -> Mem1/1, Warn/1
  Mem1/1 -> Mem2/1, Warn/2
  Mem2/1 -> Mem3/1, Warn/3
  Mem3/1 -> Mem4/1, Warn/4
  Mem4/1 -> Warn/5
  Warn/1 -> TX Warn/1

== system DR18E_Testpult/Eingabe Fahrzeug/Sensorboard Rear/Transmit OK Detection3 ==
  note: This subsystem surveys if the sending of the TX message is successful and if it meets the
      | requirements concerning the regularity of the sending.
      |
      | If for 5 consecutive execution steps the message could not be successfully sent the 'TX Warn'
      | output is set to 1. Also, the message is expected to be sent every 50 ms approximatively. If this
      | condition is not met 5 times consecutively the 'TX Warn' output is set to 1.
  TX status : Inport
  TX delta time : Inport  Port=2
  Delta time limit : Constant  Value=0.055
  Delta time limit exceeded : RelationalOperator  RndMeth=Nearest  InputSameDT=on
  Mem{1..4} (4 alike) : Memory
  OR : Logic  Operator=OR
  Prev. msg. not sent : RelationalOperator  Operator=~=  RndMeth=Nearest  InputSameDT=on
  Prev. msg. sent value : Constant
  Warn : Logic  Inputs=5
  TX Warn : Outport
  wires:
  TX delta time/1 -> Delta time limit exceeded/1
  Delta time limit/1 -> Delta time limit exceeded/2
  Prev. msg. sent value/1 -> Prev. msg. not sent/2
  TX status/1 -> Prev. msg. not sent/1
  Prev. msg. not sent/1 -> OR/1
  Delta time limit exceeded/1 -> OR/2
  OR/1 -> Mem1/1, Warn/1
  Mem1/1 -> Mem2/1, Warn/2
  Mem2/1 -> Mem3/1, Warn/3
  Mem3/1 -> Mem4/1, Warn/4
  Mem4/1 -> Warn/5
  Warn/1 -> TX Warn/1

== system DR18E_Testpult/Eingabe Fahrzeug/Sensorboard Rear/Transmit OK Detection4 ==
  note: This subsystem surveys if the sending of the TX message is successful and if it meets the
      | requirements concerning the regularity of the sending.
      |
      | If for 5 consecutive execution steps the message could not be successfully sent the 'TX Warn'
      | output is set to 1. Also, the message is expected to be sent every 50 ms approximatively. If this
      | condition is not met 5 times consecutively the 'TX Warn' output is set to 1.
  TX status : Inport
  TX delta time : Inport  Port=2
  Delta time limit : Constant  Value=0.055
  Delta time limit exceeded : RelationalOperator  RndMeth=Nearest  InputSameDT=on
  Mem{1..4} (4 alike) : Memory
  OR : Logic  Operator=OR
  Prev. msg. not sent : RelationalOperator  Operator=~=  RndMeth=Nearest  InputSameDT=on
  Prev. msg. sent value : Constant
  Warn : Logic  Inputs=5
  TX Warn : Outport
  wires:
  TX delta time/1 -> Delta time limit exceeded/1
  Delta time limit/1 -> Delta time limit exceeded/2
  Prev. msg. sent value/1 -> Prev. msg. not sent/2
  TX status/1 -> Prev. msg. not sent/1
  Prev. msg. not sent/1 -> OR/1
  Delta time limit exceeded/1 -> OR/2
  OR/1 -> Mem1/1, Warn/1
  Mem1/1 -> Mem2/1, Warn/2
  Mem2/1 -> Mem3/1, Warn/3
  Mem3/1 -> Mem4/1, Warn/4
  Mem4/1 -> Warn/5
  Warn/1 -> TX Warn/1

== system DR18E_Testpult/RTI Data/RTI Data Store/RTI Data Store ==
  RTI Data Store : Subsystem  mask(RTI_DATA_STORE){}
      mask help:
      | RTI Data Store Block. This block is used by RTI to store internal model dependent data. Deleting this block will result in data loss.
      |
      | NEVER DELETE, COPY, OR MODIFY THIS BLOCK!
      mask Help:
      | RTI Data Store Block. This block is used by RTI to store internal model dependent data. Deleting this block will result in data loss.
      | 
      | NEVER DELETE, COPY, OR MODIFY THIS BLOCK!
      mask Display: text(0.5, 0.5, ' ', 'HorizontalAlignment', 'center');

== system DR18E_Testpult/Verarbeitung/Alarme/AMSIMD_Latching ==
  AMS Error : Inport
  IMD Error : Inport  Port=2
  AMS_IMD_Reset : Inport  Port=3
  Enable : EnablePort
  S-R Flip-Flop : simulink_extras/Flip Flops/S-R Flip-Flop  initial_condition=0
  S-R Flip-Flop1 : simulink_extras/Flip Flops/S-R Flip-Flop  initial_condition=0
  AMS_ErrorOut : Outport
  IMD_ErrorOut : Outport  Port=2
  wires:
  AMS_IMD_Reset/1 -> S-R Flip-Flop/2, S-R Flip-Flop1/2
  IMD Error/1 -> S-R Flip-Flop1/1
  AMS Error/1 -> S-R Flip-Flop/1
  S-R Flip-Flop/1 -> AMS_ErrorOut/1
  S-R Flip-Flop1/1 -> IMD_ErrorOut/1

== system DR18E_Testpult/Verarbeitung/Alarme/ErrorCodeTX ==
  In : Inport
  Bus Selector : BusSelector  OutputSignals=Sicherheitskreis.A_BSPD,Sicherheitskreis.A_BRAKE_OVERTRAVEL,Sicherheitskreis.A_NOT_COCKPIT,Sicherheitskreis.A_NOT_LINKS,Sicherheitskreis.A_NOT_RECHTS,Sicherheitskreis.A_AMS_out,Sicherheitskreis.A_IMD_out,Sicherheitskreis.A_HVD,BRInplausible,GasTimeout,BremseTimeout,Gas1Status,Gas2Status,BremseVorneStatus,BremseHintenStatus,DrehzahlTimeout,LenkwinkelTimeout
  Gain : Gain
  Gain1 : Gain  Gain=2
  Gain10 : Gain  Gain=43
  Gain11 : Gain  Gain=44
  Gain12 : Gain  Gain=45
  Gain13 : Gain  Gain=46
  Gain2 : Gain  Gain=3
  Gain3 : Gain  Gain=4
  Gain4 : Gain  Gain=5
  Gain5 : Gain  Gain=6
  Gain6 : Gain  Gain=7
  Gain7 : Gain  Gain=8
  Gain8 : Gain  Gain=41
  Gain9 : Gain  Gain=42
  Logical Operator : Logic  Operator=OR  AllPortsSameDT=off  OutDataTypeStr=boolean
  Logical Operator1 : Logic  Operator=OR  AllPortsSameDT=off  OutDataTypeStr=boolean
  Logical Operator2 : Logic  Operator=OR  AllPortsSameDT=off  OutDataTypeStr=boolean
  MinMax : MinMax  Function=max  Inputs=14
  ErrorCode : Outport
  wires:
  Bus Selector/1 -> Gain/1  "<A_BSPD>"
  MinMax/1 -> ErrorCode/1
  Gain/1 -> MinMax/1
  Bus Selector/2 -> Gain1/1  "<A_BRAKE_OVERTRAVEL>"
  Gain1/1 -> MinMax/2
  Bus Selector/3 -> Gain2/1  "<A_NOT_COCKPIT>"
  Gain2/1 -> MinMax/3
  Bus Selector/4 -> Gain3/1  "<A_NOT_LINKS>"
  Gain3/1 -> MinMax/4
  Bus Selector/5 -> Gain4/1  "<A_NOT_RECHTS>"
  Gain4/1 -> MinMax/5
  Bus Selector/6 -> Gain5/1  "<A_AMS_out>"
  Gain5/1 -> MinMax/6
  Bus Selector/7 -> Gain6/1  "<A_IMD_out>"
  Gain6/1 -> MinMax/7
  Bus Selector/8 -> Gain7/1  "<A_HVD>"
  Gain7/1 -> MinMax/8
  Bus Selector/9 -> Gain8/1  "<BRInplausible>"
  Gain8/1 -> MinMax/9
  In/1 -> Bus Selector/1
  Bus Selector/10 -> Logical Operator/1  "<GasTimeout>"
  Bus Selector/11 -> Logical Operator/2  "<BremseTimeout>"
  Logical Operator/1 -> Gain9/1
  Gain9/1 -> MinMax/10
  Logical Operator1/1 -> Gain10/1
  Bus Selector/12 -> Logical Operator1/1  "<Gas1Status>"
  Bus Selector/13 -> Logical Operator1/2  "<Gas2Status>"
  Gain10/1 -> MinMax/11
  Logical Operator2/1 -> Gain11/1
  Bus Selector/14 -> Logical Operator2/1  "<BremseVorneStatus>"
  Bus Selector/15 -> Logical Operator2/2  "<BremseHintenStatus>"
  Gain11/1 -> MinMax/12
  Bus Selector/16 -> Gain12/1  "<DrehzahlTimeout>"
  Gain12/1 -> MinMax/13
  Bus Selector/17 -> Gain13/1  "<LenkwinkelTimeout>"
  Gain13/1 -> MinMax/14

== system DR18E_Testpult/Verarbeitung/Bremse/FlightRecorder ==
  In1 : Inport
  Data Type Conversion : DataTypeConversion
  Gain : Gain
  USB_FLIGHT_REC_BL1 : rtiusbflightreclib/USB_FLIGHT_REC_BL1  VarName=BremsdruckVorne  DataType=Single  SampleTime=-1  TLCFileName=rtiusbflightrecwrite  Reserved1=[]  Reserved2=[]  Reserved3=[]  Reserved4=[]  DSProperties=struct('RTI',struct('Version',uint32(3),'BlockType',struct('isSLSource',uint8(0),'isSLSink',uint8(1),'isHWSource',uint8(0),'isHWSink',uint8(0),'isSetup',uint8(0),'isInline',uint8(1),'isNonInline',uint8(0),'isInterrupt',uint8(0),'isChannelwise',uint8(0)),'IOBoardType',{{'DSUSB','FLIGHTREC'}},'UnitType','FLIGHTREC','Identifier','WRITE','DialogType','SL','BlockSet','RTIUSBFLIGHTREC','SlaveProcessor','NONE'))  RTIBlockInterface=struct('InputPortsActive',1,'InputPortsWidth',int32(1),'InputPortsDataType',{{'SS_SINGLE'}},'BlockDisplay',{{['Write to\nUSB Flight Recorder'],'center'}},'IconTransparency','off','InitLevel',3,'BlockName',struct('Token',{{'USB_FLIGHT_REC_BL1'}}),'MaskDescription',['Write input to the Flight Recorder. Recorded data can be referenced by the specified variable.'],'SampleTime',{{-1}})  RTIBlockParameters=struct('VarName',{{'BremsdruckVorne','OFF',[]}},'DataType',{{'Single','OFF',[]}},'SampleTime',{{-1,'OFF',[]}},'TLCFileName',{{'rtiusbflightrecwrite','OFF',[]}})  RTISFcnParameters=struct('VarName','char','DataType','char','SampleTime','double','TLCFileName','char')  RTIBlockParaDefault=struct('VarName','Var1','DataType','Single','SampleTime',-1,'TLCFileName','rtiusbflightrecwrite')
      settings: SourceProductName=dSPACE RTI USB Flight Rec Blockset
  wires:
  Gain/1 -> Data Type Conversion/1
  In1/1 -> Gain/1
  Data Type Conversion/1 -> USB_FLIGHT_REC_BL1/1

== system DR18E_Testpult/Verarbeitung/Bremse/FlightRecorder1 ==
  In1 : Inport
  Data Type Conversion : DataTypeConversion
  Gain : Gain
  USB_FLIGHT_REC_BL1 : rtiusbflightreclib/USB_FLIGHT_REC_BL1  VarName=BremsdruckHinten  DataType=Single  SampleTime=-1  TLCFileName=rtiusbflightrecwrite  Reserved1=[]  Reserved2=[]  Reserved3=[]  Reserved4=[]  DSProperties=struct('RTI',struct('Version',uint32(3),'BlockType',struct('isSLSource',uint8(0),'isSLSink',uint8(1),'isHWSource',uint8(0),'isHWSink',uint8(0),'isSetup',uint8(0),'isInline',uint8(1),'isNonInline',uint8(0),'isInterrupt',uint8(0),'isChannelwise',uint8(0)),'IOBoardType',{{'DSUSB','FLIGHTREC'}},'UnitType','FLIGHTREC','Identifier','WRITE','DialogType','SL','BlockSet','RTIUSBFLIGHTREC','SlaveProcessor','NONE'))  RTIBlockInterface=struct('InputPortsActive',1,'InputPortsWidth',int32(1),'InputPortsDataType',{{'SS_SINGLE'}},'BlockDisplay',{{['Write to\nUSB Flight Recorder'],'center'}},'IconTransparency','off','InitLevel',3,'BlockName',struct('Token',{{'USB_FLIGHT_REC_BL1'}}),'MaskDescription',['Write input to the Flight Recorder. Recorded data can be referenced by the specified variable.'],'SampleTime',{{-1}})  RTIBlockParameters=struct('VarName',{{'BremsdruckHinten','OFF',[]}},'DataType',{{'Single','OFF',[]}},'SampleTime',{{-1,'OFF',[]}},'TLCFileName',{{'rtiusbflightrecwrite','OFF',[]}})  RTISFcnParameters=struct('VarName','char','DataType','char','SampleTime','double','TLCFileName','char')  RTIBlockParaDefault=struct('VarName','Var1','DataType','Single','SampleTime',-1,'TLCFileName','rtiusbflightrecwrite')
      settings: SourceProductName=dSPACE RTI USB Flight Rec Blockset
  wires:
  Gain/1 -> Data Type Conversion/1
  In1/1 -> Gain/1
  Data Type Conversion/1 -> USB_FLIGHT_REC_BL1/1

== system DR18E_Testpult/Verarbeitung/Bremse/FlightRecorder2 ==
  In1 : Inport
  Data Type Conversion : DataTypeConversion
  Gain : Gain
  USB_FLIGHT_REC_BL1 : rtiusbflightreclib/USB_FLIGHT_REC_BL1  VarName=Bremse_bin  DataType=Single  SampleTime=-1  TLCFileName=rtiusbflightrecwrite  Reserved1=[]  Reserved2=[]  Reserved3=[]  Reserved4=[]  DSProperties=struct('RTI',struct('Version',uint32(3),'BlockType',struct('isSLSource',uint8(0),'isSLSink',uint8(1),'isHWSource',uint8(0),'isHWSink',uint8(0),'isSetup',uint8(0),'isInline',uint8(1),'isNonInline',uint8(0),'isInterrupt',uint8(0),'isChannelwise',uint8(0)),'IOBoardType',{{'DSUSB','FLIGHTREC'}},'UnitType','FLIGHTREC','Identifier','WRITE','DialogType','SL','BlockSet','RTIUSBFLIGHTREC','SlaveProcessor','NONE'))  RTIBlockInterface=struct('InputPortsActive',1,'InputPortsWidth',int32(1),'InputPortsDataType',{{'SS_SINGLE'}},'BlockDisplay',{{['Write to\nUSB Flight Recorder'],'center'}},'IconTransparency','off','InitLevel',3,'BlockName',struct('Token',{{'USB_FLIGHT_REC_BL1'}}),'MaskDescription',['Write input to the Flight Recorder. Recorded data can be referenced by the specified variable.'],'SampleTime',{{-1}})  RTIBlockParameters=struct('VarName',{{'Bremse_bin','OFF',[]}},'DataType',{{'Single','OFF',[]}},'SampleTime',{{-1,'OFF',[]}},'TLCFileName',{{'rtiusbflightrecwrite','OFF',[]}})  RTISFcnParameters=struct('VarName','char','DataType','char','SampleTime','double','TLCFileName','char')  RTIBlockParaDefault=struct('VarName','Var1','DataType','Single','SampleTime',-1,'TLCFileName','rtiusbflightrecwrite')
      settings: SourceProductName=dSPACE RTI USB Flight Rec Blockset
  wires:
  Gain/1 -> Data Type Conversion/1
  In1/1 -> Gain/1
  Data Type Conversion/1 -> USB_FLIGHT_REC_BL1/1

== system DR18E_Testpult/Verarbeitung/Bremse/PT1 Discrete2 ==
  u : Inport
  K : Inport  Port=2
  T : Inport  Port=3
  Memory : Memory
  Product : Product
  Product1 : Product
  Subsystem : Subsystem
  Sum : Sum  Inputs=|+-
  Sum1 : Sum  Inputs=|++
  y : Outport
  wires:
  T/1 -> Subsystem/1(T)
  Product/1 -> Sum/1
  Sum1/1 -> Memory/1, y/1
  Memory/1 -> Sum/2, Sum1/2
  Product1/1 -> Sum1/1
  Sum/1 -> Product1/2
  u/1 -> Product/2
  Subsystem/1(T*) -> Product1/1
  K/1 -> Product/1

== system DR18E_Testpult/Verarbeitung/Bremse/PlausibilityCheck ==
  note: kein Bremsdruck hinten
  note: kein Bremsdruck vorne
  Bremsdruck vorne : Inport
  Bremsdruck hinten : Inport  Port=2
  Gaspedal % : Inport  Port=3
  Bus Selector : BusSelector  OutputSignals=Throttle_1,Throttle_2
  Compare To Constant : simulink/Logic and Bit Operations/Compare To Constant  relop=>=  const=50  OutDataTypeStr=boolean
  Compare To Constant1 : simulink/Logic and Bit Operations/Compare To Constant  relop=<=  const=5  OutDataTypeStr=boolean
  Compare To Constant2 : simulink/Logic and Bit Operations/Compare To Constant  relop=<=  const=5  OutDataTypeStr=boolean
  Compare To Constant3 : simulink/Logic and Bit Operations/Compare To Constant  relop=>=  const=50  OutDataTypeStr=boolean
  Compare To Constant4 : simulink/Logic and Bit Operations/Compare To Constant  relop=>=  const=20  OutDataTypeStr=boolean
  Compare To Constant5 : simulink/Logic and Bit Operations/Compare To Constant  relop=>=  const=25  OutDataTypeStr=boolean
  Compare To Constant6 : simulink/Logic and Bit Operations/Compare To Constant  relop=>=  const=0.67  OutDataTypeStr=boolean
  Compare To Constant7 : simulink/Logic and Bit Operations/Compare To Constant  relop=<  const=5  OutDataTypeStr=boolean
  Data Type Conversion : DataTypeConversion  OutDataTypeStr=double
  KPlaus : Constant
  Logical Operator : Logic  AllPortsSameDT=off  OutDataTypeStr=boolean
  Logical Operator1 : Logic  AllPortsSameDT=off  OutDataTypeStr=boolean
  Logical Operator2 : Logic  Operator=OR  Inputs=3  AllPortsSameDT=off  OutDataTypeStr=boolean
  Logical Operator3 : Logic  AllPortsSameDT=off  OutDataTypeStr=boolean
  MinMax : MinMax  Function=max  Inputs=2
  MinMax1 : MinMax  Function=max  Inputs=2
  PT1 Discrete1 : Subsystem
  S-R Flip-Flop : simulink_extras/Flip Flops/S-R Flip-Flop  initial_condition=0
  TPlaus : Constant  Value=0.5
  W_Bremse_Inplausibel : Outport
  wires:
  Compare To Constant7/1 -> S-R Flip-Flop/2
  Logical Operator3/1 -> S-R Flip-Flop/1
  Compare To Constant6/1 -> W_Bremse_Inplausibel/1
  S-R Flip-Flop/1 -> Logical Operator2/3
  Logical Operator2/1 -> Data Type Conversion/1
  PT1 Discrete1/1(y) -> Compare To Constant6/1
  Data Type Conversion/1 -> PT1 Discrete1/1(u)
  KPlaus/1 -> PT1 Discrete1/2(K)
  TPlaus/1 -> PT1 Discrete1/3(T)
  MinMax1/1 -> Compare To Constant5/1, Compare To Constant7/1
  Bus Selector/2 -> MinMax1/2  "<Throttle_2>"
  Bus Selector/1 -> MinMax1/1  "<Throttle_1>"
  Gaspedal %/1 -> Bus Selector/1
  Compare To Constant5/1 -> Logical Operator3/2
  Compare To Constant4/1 -> Logical Operator3/1
  MinMax/1 -> Compare To Constant4/1
  Logical Operator1/1 -> Logical Operator2/2
  Logical Operator/1 -> Logical Operator2/1
  Compare To Constant3/1 -> Logical Operator1/2
  Compare To Constant2/1 -> Logical Operator1/1
  Bremsdruck hinten/1 -> Compare To Constant1/1, Compare To Constant3/1, MinMax/2
  Bremsdruck vorne/1 -> Compare To Constant/1, Compare To Constant2/1, MinMax/1
  Compare To Constant1/1 -> Logical Operator/2
  Compare To Constant/1 -> Logical Operator/1

== system DR18E_Testpult/Verarbeitung/DIS/LED Bar Blinken Subsystem ==
  LED Blinken : Inport
  LED Farbe : Inport  Port=2
  "Constant " : Constant  OutDataTypeStr=boolean
  LED aus : Constant  Value=0
  LED gelb : Constant  Value=3
  LED gruen : Constant  Value=2
  LED rot : Constant
  Multiport Switch : MultiPortSwitch  Inputs=4
  Product : Product
  Pulse Generator : DiscretePulseGenerator  PulseType=Time based  Period=1  PulseWidth=50
  Switch : Switch  Criteria=u2 > Threshold
  Out1 : Outport
  wires:
  LED aus/1 -> Multiport Switch/2  "LED aus"
  Multiport Switch/1 -> Product/2  "LED_BAR_2"
  LED rot/1 -> Multiport Switch/3  "LED rot"
  Pulse Generator/1 -> Switch/1
  Product/1 -> Out1/1
  "Constant "/1 -> Switch/3
  Switch/1 -> Product/1
  LED Blinken/1 -> Switch/2
  LED gruen/1 -> Multiport Switch/4  "LED gruen"
  LED gelb/1 -> Multiport Switch/5  "LED gelb"
  LED Farbe/1 -> Multiport Switch/1
